simulink model "simulink_1"  (R2013a)
settings: Solver=ode45  StartTime=0.0  StopTime=100  FixedStep=0.5  RelTol=1e-3
values from neighbouring files (symbols this model uses):
  L = 6.2e-3    (= 0.0062)    [Aula10_RK2.m]    (also in Aula10_RK4.m; lab6_2.m)
  R = 50    [Aula10_RK2.m]    (also in Aula10_RK4.m)
undefined symbols (not defined in the file or in its folder): CL
settings Model: Creator=43975686855  LastModifiedBy=43975686855

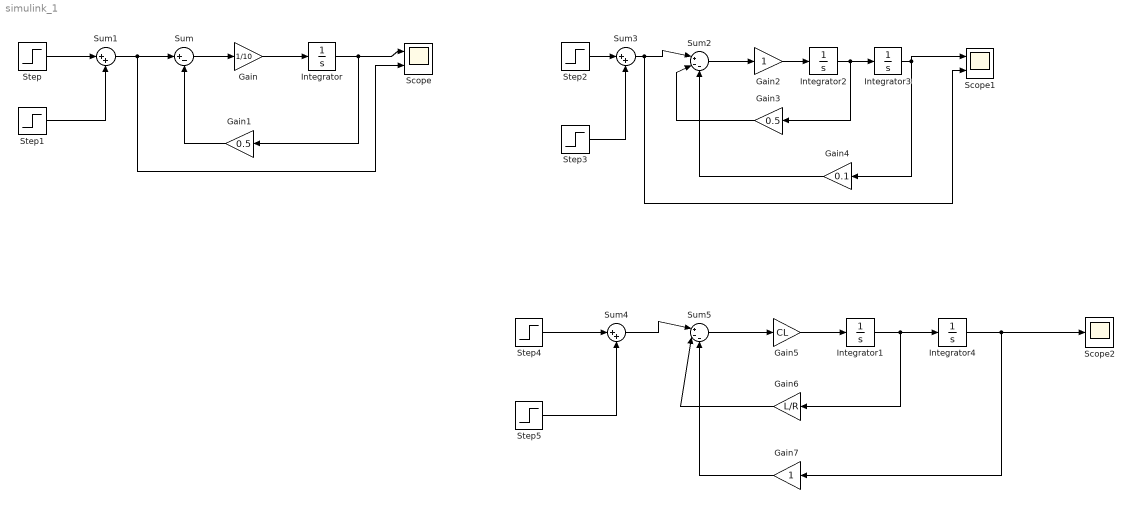
== system simulink_1 ==
  Gain : Gain  Gain=1/10
  Gain1 : Gain  Gain=0.5
  Gain2 : Gain
  Gain3 : Gain  Gain=0.5
  Gain4 : Gain  Gain=0.1
  Gain5 : Gain  Gain=CL
  Gain6 : Gain  Gain=L/R
  Gain7 : Gain
  Integrator{,1..4} (5 alike) : Integrator
  Scope : Scope  NumInputPorts=2
      settings: YMin=-5~-5  YMax=5~5
  Scope1 : Scope  NumInputPorts=2
      settings: YMin=-5~-5  YMax=5~5
  Scope2 : Scope
      settings: SaveName=ScopeData2
  Step : Step  Time=10  SampleTime=0
  Step1 : Step  Time=15  After=-1  SampleTime=0
  Step2 : Step  Time=10  SampleTime=0
  Step3 : Step  Time=15  After=-1  SampleTime=0
  Step4 : Step  Time=10  SampleTime=0
  Step5 : Step  Time=15  After=-1  SampleTime=0
  Sum : Sum  Inputs=|+-
  Sum1 : Sum  Inputs=|++
  Sum2 : Sum  Inputs=|+--
  Sum3 : Sum  Inputs=|++
  Sum4 : Sum  Inputs=|++
  Sum5 : Sum  Inputs=|+--
  wires:
  Sum/1 -> Gain/1
  Gain1/1 -> Sum/2
  Gain/1 -> Integrator/1
  Integrator/1 -> Scope/1, Gain1/1
  Step1/1 -> Sum1/2
  Step/1 -> Sum1/1
  Sum1/1 -> Scope/2, Sum/1
  Sum2/1 -> Gain2/1
  Gain2/1 -> Integrator2/1
  Integrator2/1 -> Gain3/1, Integrator3/1
  Gain3/1 -> Sum2/2
  Integrator3/1 -> Gain4/1, Scope1/1
  Gain4/1 -> Sum2/3
  Step2/1 -> Sum3/1
  Step3/1 -> Sum3/2
  Sum3/1 -> Scope1/2, Sum2/1
  Sum5/1 -> Gain5/1
  Gain5/1 -> Integrator1/1
  Integrator1/1 -> Gain6/1, Integrator4/1
  Gain6/1 -> Sum5/2
  Gain7/1 -> Sum5/3
  Integrator4/1 -> Gain7/1, Scope2/1
  Sum4/1 -> Sum5/1
  Step4/1 -> Sum4/1
  Step5/1 -> Sum4/2
